simulink model "Simulate"  (R2024b)
settings: Solver=VariableStepAuto  StartTime=0.0  StopTime=Tf  FixedStep=Ti  MaxStep=Ti  RelTol=1e-3
undefined symbols (not defined in the file): AA, AAineq, Ad_KF, BB, bbineq, C_KF, Cf, dKF_ROT, EE, H, KF, KF_ROT, lambda_u, Lf, nH, Np, nx, plecs, Rf, t_charge, Tab2abc, Tabc2ab, Ti, Ts, v_max, Vdc, Vo, w, Wx
libraries: eeTotalHarmonicDistorsion x3, simulink x1, dspstat3 x1, spsPWMGenerator3LevelLib x1
settings Model: Creator=lokit  LastModifiedBy=Pablo
settings SolverCC: InitialStep=Ti/10
settings RTWCC: GPUComputeCapability=3.5

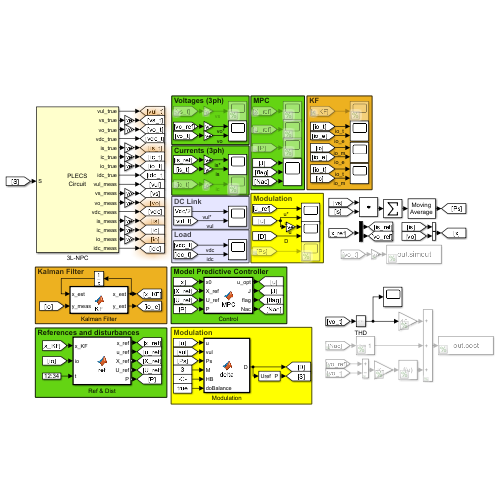
[thumbnail: Simulink's stored preview of the top-level diagram]
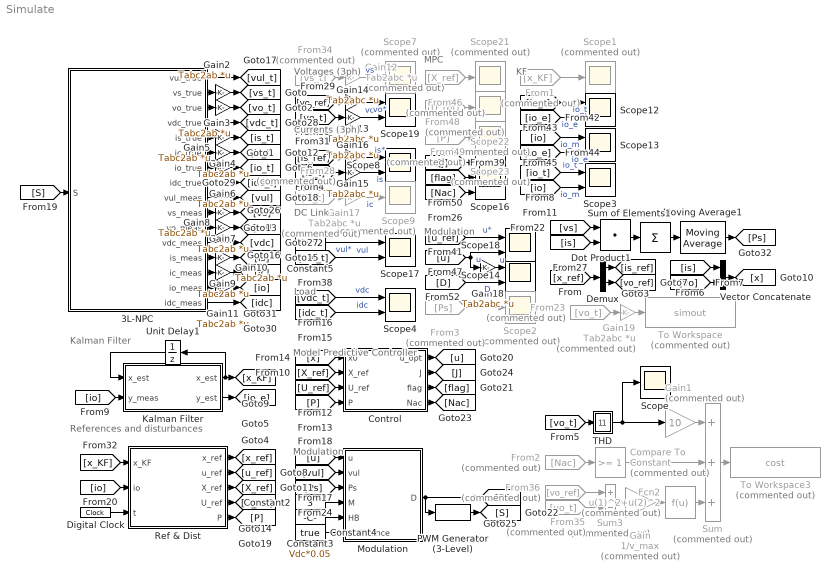
== system Simulate ==
  note: Modulation
  note: Model Predictive Controller
  note: Kalman Filter
  note: Load
  note: DC Link
  note: Modulation
  note: KF
  note: MPC
  note: Voltages (3ph)
  note: Currents (3ph)
  note: References and disturbances
  3L-NPC : Subsystem  LoadFcn=plecs('sl', 200);  InitFcn=plecs('sl', 214);  StartFcn=plecs('sl', 208);  StopFcn=plecs('sl', 209);  mask(PlecsCircuit){PLECSData=<binary blob, 9604 chars, not shown>}
      mask prompts: PLECSData "PLECS Data (Do not delete or modify!)"
      mask init:
      | % PLACE CUSTOM INITIALIZATIONS ABOVE
      | % DO NOT REMOVE
      | plecs('sl', 215);
      | % DO NOT REMOVE
      settings: CopyFcn=plecs('sl', 203);  DeleteFcn=plecs('sl', 205);  UndoDeleteFcn=plecs('sl', 206);  PreSaveFcn=plecs('sl', 211);  PostSaveFcn=plecs('sl', 201);  NameChangeFcn=plecs('sl', 210);  DestroyFcn=plecs('sl', 207);  PreCopyFcn=plecs('sl', 216);  OpenFcn=plecs('sl', 202);  ErrorFcn=plerrorfcn
      mask Help: eval('plecs(''help'', ''qthelp:///creatingacircuit.html'')')
      mask Display: disp('PLECS\nCircuit')
  Compare To Constant : simulink/Logic and Bit Operations/Compare To Constant  Commented=on  relop=>=  const=1  OutDataTypeStr=uint8
  Constant2 : Constant  Value=3  SampleTime=Ts
  Constant3 : Constant  Value=Vdc*0.05  SampleTime=Ts
  Constant4 : Constant  Value=true  OutDataTypeStr=boolean  SampleTime=Ts
  Constant5 : Constant  Value=Vdc/2  SampleTime=Ti
  Control : MATLAB Function  TreatAsAtomicUnit=on  SystemSampleTime=Ts
  Demux : Demux  Outputs=[2; 2]
  Digital Clock : DigitalClock  SampleTime=Ts
  Dot Product1 : DotProduct  OutDataTypeStr=Inherit: Inherit via internal rule
  Fcn2 : Fcn  Commented=on  Expr=u(1)^2+u(2)^2
  From1 : From  Commented=on  GotoTag=x_KF
  From2 : From  Commented=on  GotoTag=Nac
  From23 : From  Commented=on  GotoTag=vo_t
  From28 : From  Commented=on  GotoTag=ic_t
  From3 : From  Commented=on  GotoTag=Ps
  From34 : From  Commented=on  GotoTag=vs_t
  From35 : From  Commented=on  GotoTag=vo_t
  From36 : From  Commented=on  GotoTag=vo_ref
  From46 : From  Commented=on  GotoTag=X_ref
  From48 : From  Commented=on  GotoTag=U_ref
  From49 : From  Commented=on  GotoTag=P
  Gain : Gain  Commented=on  Gain=1/v_max
  Gain1 : Gain  Commented=on  Gain=10
  Gain{2..11} (10 alike) : Gain  Gain=Tabc2ab  Multiplication=Matrix(K*u) (u vector)
  Gain12 : Gain  Commented=on  Gain=Tab2abc  Multiplication=Matrix(K*u) (u vector)
  Gain{13..16,18} (5 alike) : Gain  Gain=Tab2abc  Multiplication=Matrix(K*u) (u vector)
  Gain17 : Gain  Commented=on  Gain=Tab2abc  Multiplication=Matrix(K*u) (u vector)
  Gain19 : Gain  Commented=on  Gain=Tab2abc  Multiplication=Matrix(K*u) (u vector)
  Kalman Filter : MATLAB Function  TreatAsAtomicUnit=on  SystemSampleTime=Ts
  Modulation : MATLAB Function  TreatAsAtomicUnit=on  SystemSampleTime=Ts
  Moving Average1 : dspstat3/Moving Average  Method=Sliding window  ForgettingFactorPort=off  SpecifyWindowLength=on  WindowLength=1  OverlapLength=0  AllowArbitraryInputLength=off  ForgettingFactor=0.9  SimulateUsing=Interpreted execution
  PWM Generator (3-Level) : spsPWMGenerator3LevelLib/PWM Generator (3-Level)  ModulatorType=Three-phase bridge (12 pulses)  ModulatorMode=Unsynchronized  nF=27  Fc=fc  ModulatingSignals=off  m=0.8  Freq=60  Phase=0  Ts=0
      settings: LibrarySourceBlock=|
      | sps_lib/Power Electronics/Power Electronics Control/PWM Generator
      | (3-Level)
  Ref & Dist : MATLAB Function  TreatAsAtomicUnit=on  SystemSampleTime=Ts
  Scope : Scope
  Scope{1..2,7,9,21..23} (7 alike) : Scope  Commented=on
  Scope{3..4,8,12..14,17..19} (9 alike) : Scope  NumInputPorts=2
  Scope16 : Scope  NumInputPorts=3
  Sum : Sum  Commented=on  Inputs=+++
  Sum of Elements1 : Sum  Inputs=+
  Sum3 : Sum  Commented=on  Inputs=+-
  THD : Subsystem
  To Workspace : ToWorkspace  Commented=on  VariableName=simout  SaveFormat=Timeseries  SampleTime=-1
  To Workspace3 : ToWorkspace  Commented=on  VariableName=cost  SaveFormat=Timeseries  SampleTime=Ts
  Unit Delay1 : UnitDelay  InitialCondition=zeros(nH, 1)  SampleTime=Ts  HasFrameUpgradeWarning=on
  Vector Concatenate : Concatenate
  wires:
  [is] -> Vector Concatenate/1
  [vo] -> Vector Concatenate/2
  Vector Concatenate/1 -> [x]
  Demux/1 -> [is_ref]
  [x_ref] -> Demux/1
  Demux/2 -> [vo_ref]
  [S] -> 3L-NPC/1(S)
  Kalman Filter/1(x_est) -> Unit Delay1/1, [x_KF]
  Kalman Filter/2(y_est) -> [io_e]
  [io] -> Kalman Filter/2(y_meas)
  [x] -> Control/1(x0)
  Ref & Dist/3(X_ref) -> [X_ref]
  Ref & Dist/4(U_ref) -> [U_ref]
  Ref & Dist/5(P) -> [P]
  [X_ref] -> Control/2(X_ref)
  [U_ref] -> Control/3(U_ref)
  [P] -> Control/4(P)
  Control/1(u_opt) -> [u]
  Control/3(flag) -> [flag]
  [u] -> Modulation/1(u)
  [Ps] -> Modulation/3(Ps)
  Constant3/1 -> Modulation/5(HB)
  Constant2/1 -> Modulation/4(M)
  Constant4/1 -> Modulation/6(doBalance)
  [vul] -> Modulation/2(vul)
  Modulation/1(D) -> PWM Generator (3-Level)/1, [D]
  PWM Generator (3-Level)/1 -> [S]
  Gain6/1 -> [io_t]
  Gain2/1 -> [vs_t]
  Gain4/1 -> [is_t]
  Gain3/1 -> [vo_t]
  Control/2(J) -> [J]
  [J] -> Scope16/1
  From49/1 -> Scope23/1
  [u_ref] -> Scope18/1  "u*"
  From46/1 -> Scope21/1
  [vul_t] -> Scope17/2  "vul"
  From48/1 -> Scope22/1
  [D] -> Scope14/2  "D"
  [u] -> Gain18/1, Scope18/2  "u"
  Constant5/1 -> Scope17/1  "vul*"
  [flag] -> Scope16/2
  From1/1 -> Scope1/1
  Gain18/1 -> Scope14/1  "u"
  From3/1 -> Scope2/1
  [io] -> Scope3/2  "io_m"
  [io_t] -> Scope3/1  "io_t"
  [vdc_t] -> Scope4/1  "vdc"
  [idc_t] -> Scope4/2  "idc"
  3L-NPC/1(vul_true) -> [vul_t]
  3L-NPC/4(vdc_true) -> [vdc_t]
  3L-NPC/8(idc_true) -> [idc_t]
  3L-NPC/2(vs_true) -> Gain2/1
  3L-NPC/3(vo_true) -> Gain3/1
  3L-NPC/5(is_true) -> Gain4/1
  3L-NPC/7(io_true) -> Gain6/1
  Gain5/1 -> [ic_t]
  3L-NPC/6(ic_true) -> Gain5/1
  3L-NPC/15(io_meas) -> Gain11/1
  Gain10/1 -> [ic]
  3L-NPC/14(ic_meas) -> Gain10/1
  3L-NPC/12(vdc_meas) -> [vdc]
  3L-NPC/16(idc_meas) -> [idc]
  3L-NPC/11(vo_meas) -> Gain8/1
  3L-NPC/13(is_meas) -> Gain9/1
  3L-NPC/10(vs_meas) -> Gain7/1
  Gain7/1 -> [vs]
  Gain11/1 -> [io]
  Gain8/1 -> [vo]
  Gain9/1 -> [is]
  3L-NPC/9(vul_meas) -> [vul]
  Gain12/1 -> Scope7/1  "vs"
  Gain14/1 -> Scope19/2  "vo"
  Gain13/1 -> Scope19/1  "vo*"
  Gain15/1 -> Scope8/1  "is*"
  Gain16/1 -> Scope8/2  "is"
  Gain17/1 -> Scope9/1  "ic"
  [is_ref] -> Gain15/1
  [vo_t] -> THD/1(In1)
  From28/1 -> Gain17/1
  From34/1 -> Gain12/1
  [vo_ref] -> Gain13/1
  [vo_t] -> Gain14/1
  Sum of Elements1/1 -> Moving Average1/1
  Moving Average1/1 -> [Ps]
  Dot Product1/1 -> Sum of Elements1/1
  [is] -> Dot Product1/2
  [vs] -> Dot Product1/1
  Unit Delay1/1 -> Kalman Filter/1("x_est ")
  Ref & Dist/1(x_ref) -> [x_ref]
  Ref & Dist/2(u_ref) -> [u_ref]
  From2/1 -> Compare To Constant/1
  Control/4(Nac) -> [Nac]
  [Nac] -> Scope16/3
  From35/1 -> Sum3/2
  From36/1 -> Sum3/1
  Sum3/1 -> Gain/1
  Gain/1 -> Fcn2/1
  [is_t] -> Gain16/1
  THD/1(Out1) -> Scope/1, Gain1/1
  From23/1 -> Gain19/1
  Gain19/1 -> To Workspace/1
  [x_KF] -> Ref & Dist/1(x_KF)
  [io_t] -> Scope12/1  "io_t"
  [io_e] -> Scope12/2  "io_e"
  [io] -> Scope13/1  "io_m"
  [io_e] -> Scope13/2  "io_e"
  Gain1/1 -> Sum/1
  Compare To Constant/1 -> Sum/2
  Fcn2/1 -> Sum/3
  Sum/1 -> To Workspace3/1
  Digital Clock/1 -> Ref & Dist/3(t)
  [io] -> Ref & Dist/2(io)

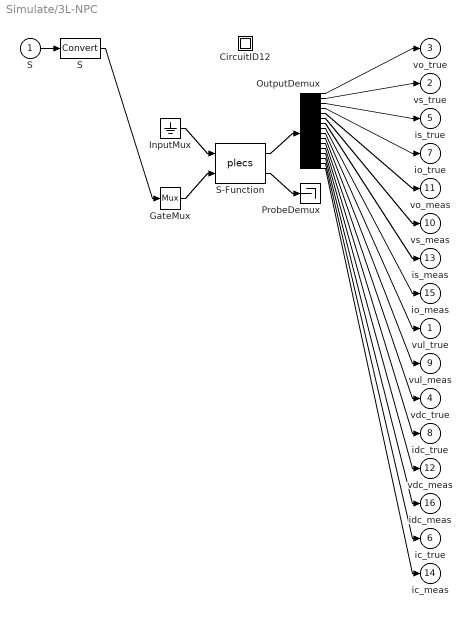
== system Simulate/3L-NPC ==
  S : Inport  PortDimensions=12
  " CircuitID12 " : Subsystem
  " GateMux " : Mux  Inputs=[ 12 ]
  " InputMux " : Ground
  " OutputDemux " : Demux  Outputs=[ 3 3 3 3 3 3 3 3 2 2 1 1 1 1 3 3 ]
  " ProbeDemux " : Terminator
  " S " : DataTypeConversion
  " S-Function " : S-Function  FunctionName=plecs  SFunctionDeploymentMode=off  EnableBusSupport=off
  vul_true : Outport  PortDimensions=2
  vs_true : Outport  Port=2  PortDimensions=3
  vo_true : Outport  Port=3  PortDimensions=3
  vdc_true : Outport  Port=4  PortDimensions=1
  is_true : Outport  Port=5  PortDimensions=3
  ic_true : Outport  Port=6  PortDimensions=3
  io_true : Outport  Port=7  PortDimensions=3
  idc_true : Outport  Port=8  PortDimensions=1
  vul_meas : Outport  Port=9  PortDimensions=2
  vs_meas : Outport  Port=10  PortDimensions=3
  vo_meas : Outport  Port=11  PortDimensions=3
  vdc_meas : Outport  Port=12  PortDimensions=1
  is_meas : Outport  Port=13  PortDimensions=3
  ic_meas : Outport  Port=14  PortDimensions=3
  io_meas : Outport  Port=15  PortDimensions=3
  idc_meas : Outport  Port=16  PortDimensions=1
  wires:
  " InputMux "/1 -> " S-Function "/1
  " GateMux "/1 -> " S-Function "/2
  " S-Function "/1 -> " OutputDemux "/1
  " S-Function "/2 -> " ProbeDemux "/1
  S/1 -> " S "/1
  " S "/1 -> " GateMux "/1
  " OutputDemux "/1 -> vo_true/1
  " OutputDemux "/2 -> vs_true/1
  " OutputDemux "/3 -> is_true/1
  " OutputDemux "/4 -> io_true/1
  " OutputDemux "/5 -> vo_meas/1
  " OutputDemux "/6 -> vs_meas/1
  " OutputDemux "/7 -> is_meas/1
  " OutputDemux "/8 -> io_meas/1
  " OutputDemux "/9 -> vul_true/1
  " OutputDemux "/10 -> vul_meas/1
  " OutputDemux "/11 -> vdc_true/1
  " OutputDemux "/12 -> idc_true/1
  " OutputDemux "/13 -> vdc_meas/1
  " OutputDemux "/14 -> idc_meas/1
  " OutputDemux "/15 -> ic_true/1
  " OutputDemux "/16 -> ic_meas/1

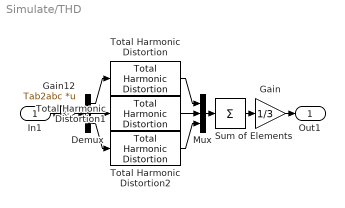
== system Simulate/THD ==
  In1 : Inport
  Demux : Demux  Outputs=3
  Gain : Gain  Gain=1/3
  Gain12 : Gain  Gain=Tab2abc  Multiplication=Matrix(K*u) (u vector)
  Mux : Mux  Inputs=3
  Sum of Elements : Sum  Inputs=+
  Total Harmonic Distortion : eeTotalHarmonicDistorsion/Total Harmonic Distortion  f=f  Ts=Ts
      settings: LibrarySourceBlock=|
      | ee_sl_lib/Measurements/Total Harmonic
      | Distortion
  Total Harmonic Distortion1 : eeTotalHarmonicDistorsion/Total Harmonic Distortion  f=f  Ts=-1
      settings: LibrarySourceBlock=|
      | ee_sl_lib/Measurements/Total Harmonic
      | Distortion
  Total Harmonic Distortion2 : eeTotalHarmonicDistorsion/Total Harmonic Distortion  f=f  Ts=-1
      settings: LibrarySourceBlock=|
      | ee_sl_lib/Measurements/Total Harmonic
      | Distortion
  Out1 : Outport
  wires:
  In1/1 -> Gain12/1
  Gain12/1 -> Demux/1
  Demux/2 -> Total Harmonic Distortion1/1
  Demux/1 -> Total Harmonic Distortion/1
  Demux/3 -> Total Harmonic Distortion2/1
  Sum of Elements/1 -> Gain/1
  Mux/1 -> Sum of Elements/1
  Total Harmonic Distortion/1 -> Mux/1
  Total Harmonic Distortion1/1 -> Mux/2
  Total Harmonic Distortion2/1 -> Mux/3
  Gain/1 -> Out1/1

== system Simulate/3L-NPC/ CircuitID12  ==

== matlab function Simulate/Kalman Filter ==
  data: x_est input; x_est output size=[nH, 1]; y_meas input size=[np, 1]; Ad_KF parameter; C_KF parameter; KF parameter; y_est output size=[np, 1]
function [x_est, y_est] = KF(x_est, y_meas, Ad_KF, C_KF, KF)

y_est = C_KF * x_est;
x_est = Ad_KF * x_est + KF * (y_meas - y_est);
y_est = C_KF * x_est;

== matlab function Simulate/Modulation ==
  data: u input; vul input; Ps input; D output; M input; HB input; doBalance input
function D = delta(u, vul, Ps, M, HB, doBalance)

% u: Converter voltage reference, normalized by xi*Vdc
% vul: Upper and lower capacitor voltages measurements
% Ps: 

%% Generalized PWM Method
vx = u(1);
vy = u(2);
theta = mod(angle(vx + 1j * vy), 2*pi);

N = floor(3 * theta / pi); % With theta = 2*pi, N = floor(6) = 6
N = N - (6 == N); % If N = 6, N = 6 - 1 = 5

fx = vx;
fy = vy / sqrt(3);

n1 = N;
n2 = 3.5 - sign(fx + 3 * fy) * ((fx > 0) + (fx > 3 * fy) + 0.5);

switch(M)
    case 1
        delta = 1;
    case 2
        delta = 0;
    case 3
        delta = 0.5;
    case 4
        delta = 0.5 * (1 + (-1)^n1);
    case 5
        delta = 0.5 * (1 + (-1)^n2);
    case 6
        delta = 0.5 * (1 + (-1)^(n1 + 1));
    case 7
        delta = 0.5 * (1 + (-1)^(n2 + 1));
    % case 8
    %     a = exp(1j * 2 * pi / 3);
    %     vr = (vx + 1j * vy) * a^(-pi / 3 * n1);
    %     vrx = real(vr);
    %     vry = imag(vr);
    %     delta = ((2 / 3 * vrx - 0.5) / (vrx + vry/sqrt(3) - 1) - 0.5) * (-1)^n1 + 0.5;
    otherwise
        error('Invalid modulation selected, M = %d', M)
end

switch(N)
    case 0
        Da = delta * (fx + fy - 1) + 1;
        Db = Da - fx + fy;
        Dc = Da - fx - fy;
    case 1
        Db = delta * (2 * fy - 1) + 1;
        Da = Db + fx - fy;
        Dc = Db - 2 * fy;
    case 2
        Db = delta * (-fx + fy - 1) + 1;
        Da = Db + fx - fy;
        Dc = Db - 2 * fy;
    case 3
        Dc = delta * (-fx - fy - 1) + 1;
        Da = Dc + fx + fy;
        Db = Dc + 2 * fy;
    case 4
        Dc = delta * (-2 * fy - 1) + 1;
        Da = Dc + fx + fy;
        Db = Dc + 2 * fy;
    case 5
        Da = delta * (fx - fy - 1) + 1;
        Db = Da - fx + fy;
        Dc = Da - fx - fy;
    otherwise
        error('Invalid modulation sector, N = %d', N)
end

D = [Da; Db; Dc];

%% Simple Capacitor Voltage Balancing
if doBalance
    vu = vul(1);
    vl = vul(2);
    if abs(vu - vl) >= HB
        if Ps >= 0
            if vu >= vl
                D = D + 1 - max(D);
            else
                D = D - 0 - min(D);
                % D = D - 1 - min(D);
            end
        else
            if vu >= vl
                D = D - 0 - min(D);
                % D = D - 1 - min(D);
            else
                D = D + 1 - max(D);
            end
        end
    end
end

D = 2 * D - 1;

== matlab function Simulate/Ref & Dist ==
  data: x_ref output; u_ref output; X_ref output; x_KF input; io input; t input; U_ref output; P output; KF_ROT parameter; dKF_ROT parameter; Vo parameter; w parameter; Rf parameter; Lf parameter; Cf parameter; Vdc parameter; Ts parameter; Np parameter; nx parameter; t_charge parameter
function [x_ref, u_ref, X_ref, U_ref, P] = ref(x_KF, io, t, KF_ROT, dKF_ROT, Vo, w, Rf, Lf, Cf, Vdc, Ts, Np, nx, t_charge)

persistent g
if isempty(g)
    g = 0;
end

% Predict disturbances
P   = KF_ROT * x_KF;
dP  = dKF_ROT * x_KF;
P(1:2) = io;
io  = P;
dio = dP;

if t < t_charge
    Vo = Vo * t / t_charge;
    w  = 0;
end

% Generate current and voltage references
g_vec = g + w*Ts*(0:Np-1);

cos_g          = cos(g_vec);
sin_g          = sin(g_vec);
cs_g           = zeros(2*Np, 1);
cs_g(1:2:end)  = cos_g;
cs_g(2:2:end)  = sin_g;
dcs_g          = zeros(2*Np, 1);
dcs_g(1:2:end) = -sin_g;
dcs_g(2:2:end) = cos_g;

is_ref = w * Cf * Vo * dcs_g + io;
vo_ref = Vo * cs_g;

X_ref          = zeros(nx*Np, 1);
X_ref(1:4:end) = is_ref(1:2:end);
X_ref(2:4:end) = is_ref(2:2:end);
X_ref(3:4:end) = vo_ref(1:2:end);
X_ref(4:4:end) = vo_ref(2:2:end);
x_ref = X_ref(1:4);

U_ref = 3*Vo/Vdc * ((1-w^2*Lf*Cf) * cs_g + w*Rf*Cf * dcs_g) + 3/Vdc * (Lf * dio + Rf * io);
U_ref = U_ref / 2;
u_ref = U_ref(1:2);

g = mod(g + w*Ts, 2*pi);

== matlab function Simulate/Control ==
  data: x0 input; X_ref input; U_ref input; P input; AA parameter; BB parameter; EE parameter; H parameter; Wx parameter; lambda_u parameter; u_opt output; J output; AAineq parameter; bbineq parameter; flag output; Nac output
function [u_opt, J, flag, Nac] = MPC(x0, X_ref, U_ref, P, AA, BB, EE, H, Wx, lambda_u, AAineq, bbineq)

persistent iA options
if isempty(iA)
    iA = false(size(AAineq, 1), 1);
    options                     = mpcActiveSetOptions;
    options.MaxIterations       = 20;
    options.ConstraintTolerance = 1e-4;
end

fx = (Wx * BB).' * (-X_ref + AA * x0 + EE * P);
fu = -2 * U_ref;
f  = fx + lambda_u * fu;

[U_opt, flag, iA, ~] = mpcActiveSetSolver(H, f, AAineq, bbineq, zeros(0, size(H, 2)), zeros(0, 1), iA, options);
Nac = sum(iA);

u_opt = U_opt(1:2);

X_pred = AA * x0 + BB * U_opt + EE * P;
Jx = (X_ref - X_pred).' * Wx * (X_ref - X_pred);
Ju = (U_ref - U_opt).' * (U_ref - U_opt);
J = Jx + lambda_u * Ju;
